simulink subsystem "Environment_Model"  (R2024b)
settings: Solver=VariableStepAuto  StartTime=0.0  StopTime=10.0  RelTol=1e-3
undefined symbols (not defined in the file or in its folder): Earth, F, Light, location, MIL, time_idle, WGS84, wind_const_direction, wind_const_strength, wind_dist_enable, wind_gust1_distribution, wind_gust1_start, wind_gust2_distribution, wind_gust2_start
libraries: aerolibwind2 x3, aerolibatmos2 x1, aerolibtransform2 x1
settings Model: Creator=joedo  LastModifiedBy=finnb

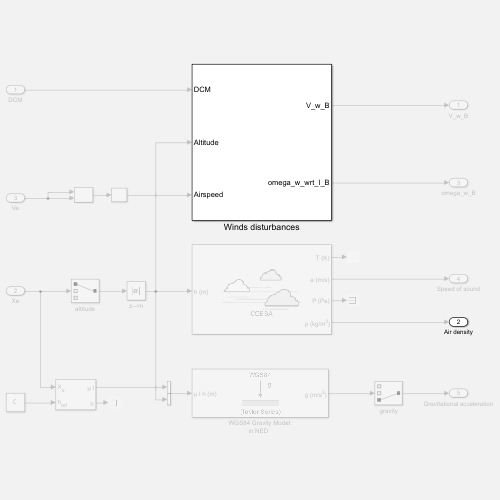
[thumbnail: Simulink's stored preview of the top-level diagram]
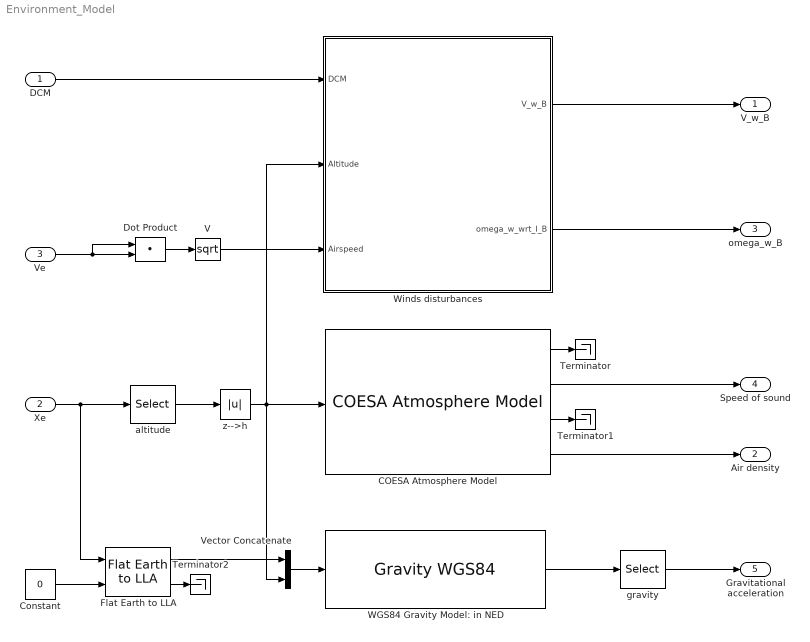
== system Environment_Model ==
  DCM : Inport
  Xe : Inport  Port=2
  Ve : Inport  Port=3
  COESA Atmosphere Model : aerolibatmos2/COESA Atmosphere Model  units=Metric (MKS)  spec=1976 COESA-extended U.S. Standard Atmosphere  model=Profile  profile_var=High temperature  profile_percent=10%  profile_alt=5 km (16404 ft)  envelope_var=High temperature  envelope_percent=1%  action=None
  Constant : Constant  Value=0
  Dot Product : DotProduct  SaturateOnIntegerOverflow=on  InputSameDT=off  OutDataTypeStr=Inherit: Inherit via internal rule
  Flat Earth to LLA : aerolibtransform2/Flat Earth to LLA  units=Metric (MKS)  ptype=Earth (WGS84)  F=1/298.257223563  R=6378137  refPosPort=off  LL0=location(2:3)  psi=0
  Terminator : Terminator
  Terminator1 : Terminator
  Terminator2 : Terminator
  V : Math  Operator=sqrt  SignedPower=on
  Vector Concatenate : Concatenate
  "WGS84 Gravity Model: in NED  " : GravityWGS84  action=Error
  Winds disturbances : Subsystem
  altitude : Selector  InputPortWidth=3  IndexOptions=Index vector (dialog)  Indices=[1]  OutputSizes=1
  gravity : Selector  InputPortWidth=3  IndexOptions=Index vector (dialog)  Indices=[3]  OutputSizes=1
  z-->h : Abs
  V_w_B : Outport  VectorParamsAs1DForOutWhenUnconnected=off
  Air density : Outport  Port=2  VectorParamsAs1DForOutWhenUnconnected=off
  omega_w_B : Outport  Port=3  VectorParamsAs1DForOutWhenUnconnected=off
  Speed of sound : Outport  Port=4  VectorParamsAs1DForOutWhenUnconnected=off
  Gravitational acceleration : Outport  Port=5
  wires:
  z-->h/1 -> Vector Concatenate/2, Winds disturbances/2(Altitude), COESA Atmosphere Model/1
  Winds disturbances/2(omega_w_wrt_I_B) -> omega_w_B/1
  DCM/1 -> Winds disturbances/1(DCM)
  Ve/1 -> Dot Product/2, Dot Product/1
  Dot Product/1 -> V/1
  V/1 -> Winds disturbances/3(Airspeed)
  COESA Atmosphere Model/2 -> Speed of sound/1
  COESA Atmosphere Model/3 -> Terminator1/1
  COESA Atmosphere Model/1 -> Terminator/1
  COESA Atmosphere Model/4 -> Air density/1
  altitude/1 -> z-->h/1
  Xe/1 -> altitude/1, Flat Earth to LLA/1
  "WGS84 Gravity Model: in NED  "/1 -> gravity/1
  Constant/1 -> Flat Earth to LLA/2
  Flat Earth to LLA/1 -> Vector Concatenate/1
  Vector Concatenate/1 -> "WGS84 Gravity Model: in NED  "/1
  gravity/1 -> Gravitational acceleration/1
  Winds disturbances/1(V_w_B) -> V_w_B/1
  Flat Earth to LLA/2 -> Terminator2/1

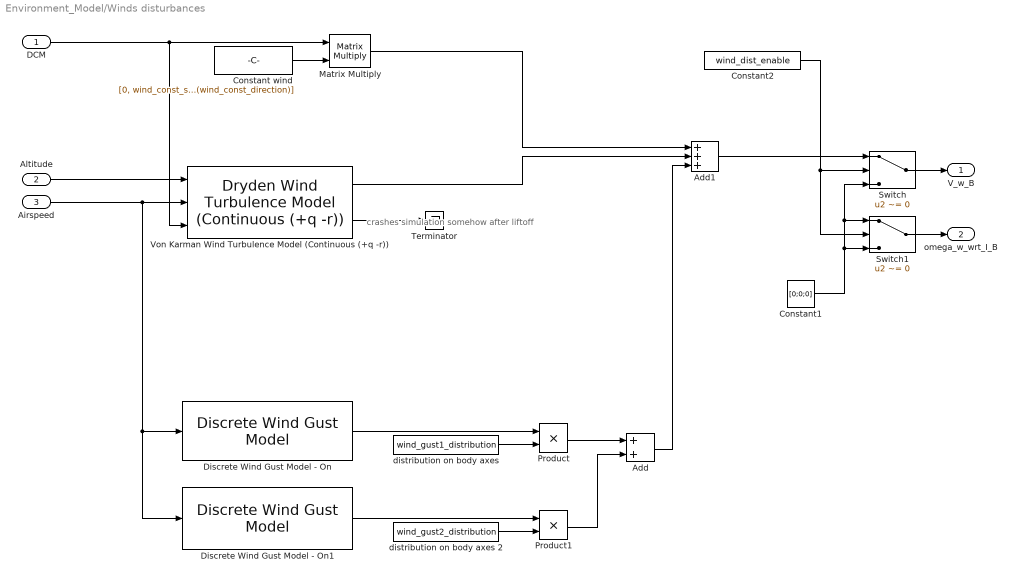
== system Environment_Model/Winds disturbances ==
  note: crashes simulation somehow after liftoff
  DCM : Inport
  Altitude : Inport  Port=2
  Airspeed : Inport  Port=3
  Add : Sum
  Add1 : Sum  Inputs=+++
  Constant wind : Constant  Value=[0, wind_const_strength*cos(wind_const_direction), wind_const_strength*sin(wind_const_direction)]
  Constant1 : Constant  Value=[0;0;0]
  Constant2 : Constant  Value=wind_dist_enable
  Discrete Wind Gust Model - On : aerolibwind2/Discrete Wind Gust Model  units=Metric (MKS)  Gx=on  Gy=on  Gz=on  t_0=time_idle + wind_gust1_start  d_m=wind_gust1_length  v_m=wind_gust1_amplitude
  Discrete Wind Gust Model - On1 : aerolibwind2/Discrete Wind Gust Model  units=Metric (MKS)  Gx=on  Gy=on  Gz=on  t_0=time_idle + wind_gust2_start  d_m=wind_gust2_length  v_m=wind_gust2_amplitude
  Matrix Multiply : Product  Multiplication=Matrix(*)
  Product : Product
  Product1 : Product
  Switch : Switch  Criteria=u2 ~= 0  SaturateOnIntegerOverflow=off  InputSameDT=off
  Switch1 : Switch  Criteria=u2 ~= 0  SaturateOnIntegerOverflow=off  InputSameDT=off
  Terminator : Terminator
  Von Karman Wind Turbulence Model (Continuous (+q -r)) : aerolibwind2/Dryden Wind Turbulence Model  (Continuous (+q -r))  units=Metric (MKS)  spec=MIL-F-8785C  model=Discrete Dryden (+q -r)  W20=wind_const_strength  Wdeg=wind_const_direction  TurbProb=10^-2 - Light  L_high=762  Wingspan=rocket_length  ts=0.1  Seed=[245341 2342 243 234]  T_on=on
  distribution on body axes : Constant  Value=wind_gust1_distribution
  distribution on body axes 2 : Constant  Value=wind_gust2_distribution
  V_w_B : Outport  VectorParamsAs1DForOutWhenUnconnected=off
  omega_w_wrt_I_B : Outport  Port=2  VectorParamsAs1DForOutWhenUnconnected=off
  wires:
  Product1/1 -> Add/2
  Product/1 -> Add/1
  Add/1 -> Add1/3
  distribution on body axes 2/1 -> Product1/2
  Discrete Wind Gust Model - On1/1 -> Product1/1
  distribution on body axes/1 -> Product/2
  Constant1/1 -> Switch/3, Switch1/1, Switch1/3
  Switch1/1 -> omega_w_wrt_I_B/1
  Constant2/1 -> Switch/2, Switch1/2
  Switch/1 -> V_w_B/1
  Add1/1 -> Switch/1
  Matrix Multiply/1 -> Add1/1
  Von Karman Wind Turbulence Model (Continuous (+q -r))/1 -> Add1/2
  Altitude/1 -> Von Karman Wind Turbulence Model (Continuous (+q -r))/1
  Airspeed/1 -> Discrete Wind Gust Model - On/1, Discrete Wind Gust Model - On1/1, Von Karman Wind Turbulence Model (Continuous (+q -r))/2
  DCM/1 -> Von Karman Wind Turbulence Model (Continuous (+q -r))/3, Matrix Multiply/1
  Discrete Wind Gust Model - On/1 -> Product/1
  Constant wind/1 -> Matrix Multiply/2
  Von Karman Wind Turbulence Model (Continuous (+q -r))/2 -> Terminator/1
